simulink model "Cabinet_D"  (Simulink 7.6)
settings: Solver=ode45  StartTime=0.0  StopTime=1000  RelTol=1e-3
values from neighbouring files (symbols this model uses):
  R = 25    [ParametersCabinet_D.m]
  sb = 5.67*(10^-8)    (= 5.67e-08)    [ParametersCabinet_D.m]
  T_amb = 296    [ParametersCabinet_D.m]
undefined symbols (not defined in the file or in its folder): CNC, Job, magnitude
libraries: simulink x1
settings Model: Creator=conid  LastModifiedBy=conid

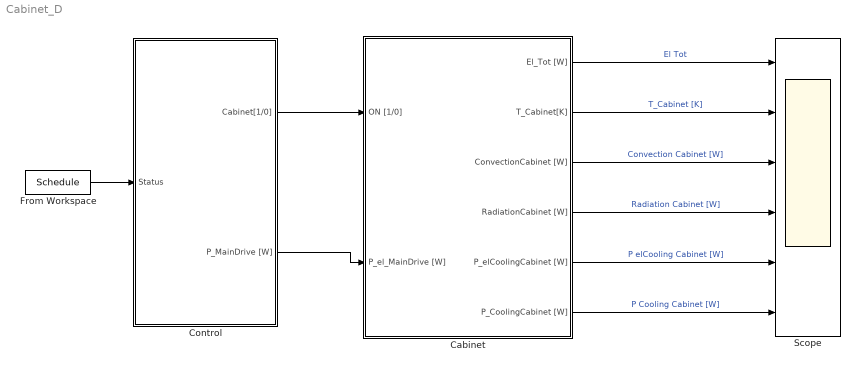
== system Cabinet_D ==
  Cabinet : Subsystem  TreatAsAtomicUnit=on
  Control : Subsystem  TreatAsAtomicUnit=on  mask{Cabinet=[0 1 1 1 1], Job=Job}
      mask prompts: Job "Job Struct"
      mask help:
      | Controls the components of the machine:
      |
      | Status:
      |     0. Off
      |     1. Standby
      |     2. Warmup
      |     3. Setting
      |     4. Machining
      |
      | If the status is machining, the job defined as
      |     - Job.time
      |     - Job.omega_dem
      |     - Job.M_dem
      | will be runned, and repeated.
      mask TabNameString: Status,Job
  From Workspace : FromWorkspace  VariableName=Schedule  SampleTime=0  Interpolate=off  OutputAfterFinalValue=Holding final value
  Scope : Scope  NumInputPorts=6
      settings: YMin=-5~-5~-5~-5~-5~-5  YMax=5~5~5~5~5~5  SaveName=Scp_Cabinet
  wires:
  Cabinet/1(El_Tot [W]) -> Scope/1  "El Tot"
  Cabinet/2(T_Cabinet[K]) -> Scope/2  "T_Cabinet [K]"
  Cabinet/3(ConvectionCabinet [W]) -> Scope/3  "Convection Cabinet [W]"
  Cabinet/4(RadiationCabinet [W]) -> Scope/4  "Radiation Cabinet [W]"
  Cabinet/5(P_elCoolingCabinet [W]) -> Scope/5  "P elCooling Cabinet [W]"
  Cabinet/6(P_CoolingCabinet [W]) -> Scope/6  "P Cooling Cabinet [W]"
  From Workspace/1 -> Control/1(Status)
  Control/1(Cabinet[1/0]) -> Cabinet/1(ON [1/0])
  Control/2(P_MainDrive [W]) -> Cabinet/2(P_el_MainDrive [W])

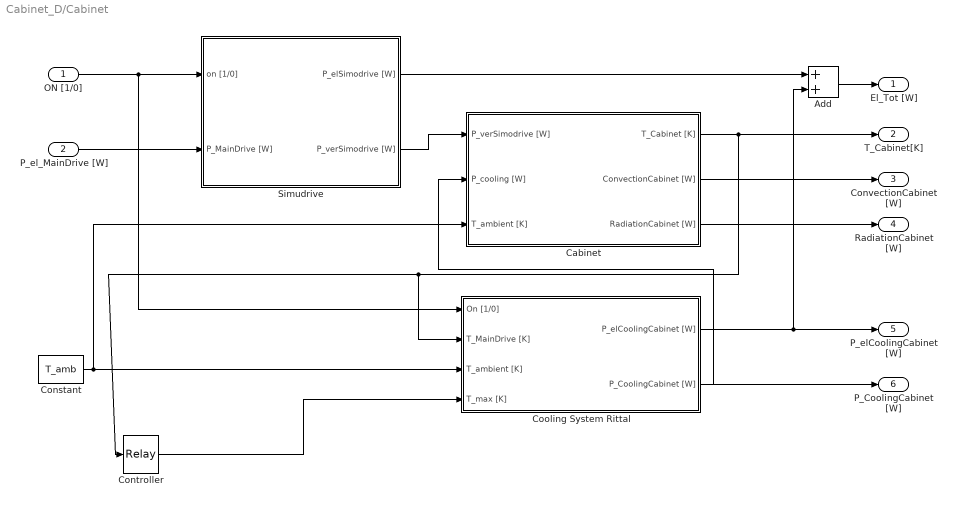
== system Cabinet_D/Cabinet ==
  ON [1/0] : Inport
  P_el_MainDrive [W] : Inport  Port=2
  Add : Sum
  Cabinet : Subsystem
  Constant : Constant  Value=T_amb
  Controller : Relay  OnSwitchValue=CNC.Cooling.Tmax  OffSwitchValue=CNC.Cooling.Tmin
  Cooling System Rittal : Subsystem
  Simudrive : Subsystem
  El_Tot [W] : Outport
  T_Cabinet[K] : Outport  Port=2
  ConvectionCabinet [W] : Outport  Port=3
  RadiationCabinet [W] : Outport  Port=4
  P_elCoolingCabinet [W] : Outport  Port=5
  P_CoolingCabinet [W] : Outport  Port=6
  wires:
  Cabinet/1(T_Cabinet [K]) -> Controller/1, Cooling System Rittal/2(T_MainDrive [K]), T_Cabinet[K]/1
  Constant/1 -> Cooling System Rittal/3(T_ambient [K]), Cabinet/3(T_ambient [K])
  Cooling System Rittal/2(P_CoolingCabinet [W]) -> Cabinet/2(P_cooling [W]), P_CoolingCabinet [W]/1
  Cabinet/2(ConvectionCabinet [W]) -> ConvectionCabinet [W]/1
  Cabinet/3(RadiationCabinet [W]) -> RadiationCabinet [W]/1
  Cooling System Rittal/1(P_elCoolingCabinet [W]) -> P_elCoolingCabinet [W]/1, Add/2
  P_el_MainDrive [W]/1 -> Simudrive/2(P_MainDrive [W])
  ON [1/0]/1 -> Simudrive/1(on [1/0]), Cooling System Rittal/1(On [1/0])
  Simudrive/2(P_verSimodrive [W]) -> Cabinet/1(P_verSimodrive [W])
  Simudrive/1(P_elSimodrive [W]) -> Add/1
  Controller/1 -> Cooling System Rittal/4(T_max [K])
  Add/1 -> El_Tot [W]/1

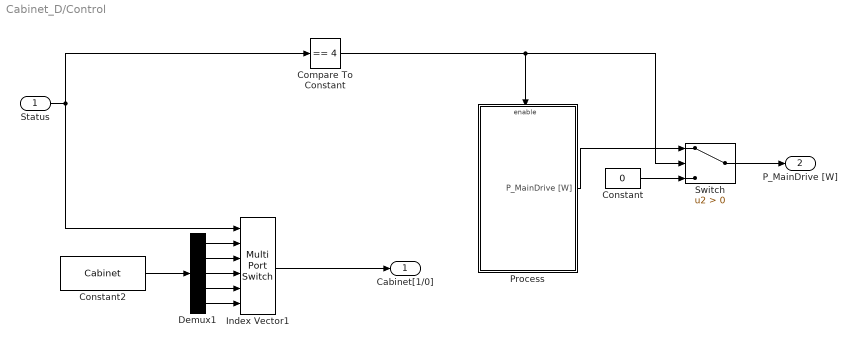
== system Cabinet_D/Control ==
  Status : Inport
  Compare To Constant : simulink/Logic and Bit Operations/Compare To Constant  SystemSampleTime=-1  relop===  const=4  LogicOutDataTypeMode=uint8
  Constant : Constant  Value=0
  Constant2 : Constant  Value=Cabinet
  Demux1 : Demux  Outputs=5
  Index Vector1 : MultiPortSwitch  DataPortOrder=Zero-based contiguous  Inputs=5  zeroidx=on
  Process : Subsystem  TreatAsAtomicUnit=on
  Switch : Switch  Criteria=u2 > Threshold
  Cabinet[1/0] : Outport
  P_MainDrive [W] : Outport  Port=2
  wires:
  Status/1 -> Compare To Constant/1, Index Vector1/1
  Demux1/1 -> Index Vector1/2
  Demux1/2 -> Index Vector1/3
  Demux1/3 -> Index Vector1/4
  Demux1/4 -> Index Vector1/5
  Demux1/5 -> Index Vector1/6
  Index Vector1/1 -> Cabinet[1/0]/1
  Compare To Constant/1 -> Process/Enable, Switch/2
  Process/1(P_MainDrive [W]) -> Switch/1
  Constant/1 -> Switch/3
  Switch/1 -> P_MainDrive [W]/1
  Constant2/1 -> Demux1/1

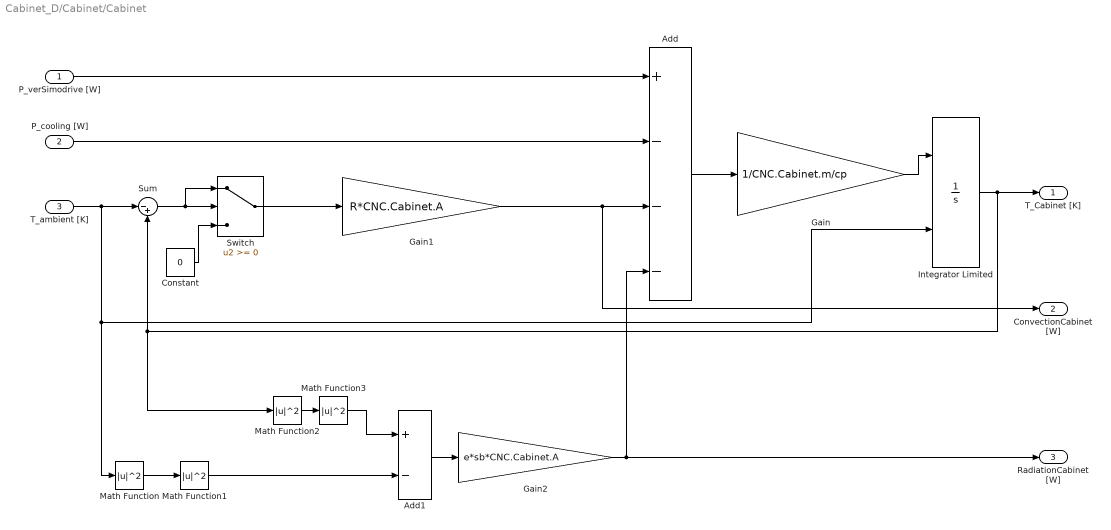
== system Cabinet_D/Cabinet/Cabinet ==
  P_verSimodrive [W] : Inport
  P_cooling [W] : Inport  Port=2
  T_ambient [K] : Inport  Port=3
  Add : Sum  Inputs=+---
  Add1 : Sum  Inputs=+-
  Constant : Constant  Value=0
  Gain : Gain  Gain=1/CNC.Cabinet.m/cp
  Gain1 : Gain  Gain=R*CNC.Cabinet.A
  Gain2 : Gain  Gain=e*sb*CNC.Cabinet.A
  Integrator Limited : Integrator  InitialConditionSource=external  LimitOutput=on
  Math Function{,1..3} (4 alike) : Math  Operator=magnitude^2  SaturateOnIntegerOverflow=on
  Sum : Sum  Inputs=|-+
  Switch : Switch
  T_Cabinet [K] : Outport
  ConvectionCabinet [W] : Outport  Port=2
  RadiationCabinet [W] : Outport  Port=3
  wires:
  P_verSimodrive [W]/1 -> Add/1
  Gain/1 -> Integrator Limited/1
  Gain1/1 -> ConvectionCabinet [W]/1, Add/3
  Integrator Limited/1 -> T_Cabinet [K]/1, Sum/2, Math Function2/1
  Add/1 -> Gain/1
  Math Function/1 -> Math Function1/1
  Gain2/1 -> RadiationCabinet [W]/1, Add/4
  P_cooling [W]/1 -> Add/2
  T_ambient [K]/1 -> Sum/1, Integrator Limited/2, Math Function/1
  Sum/1 -> Switch/2, Switch/1
  Constant/1 -> Switch/3
  Math Function2/1 -> Math Function3/1
  Add1/1 -> Gain2/1
  Math Function3/1 -> Add1/1
  Math Function1/1 -> Add1/2
  Switch/1 -> Gain1/1

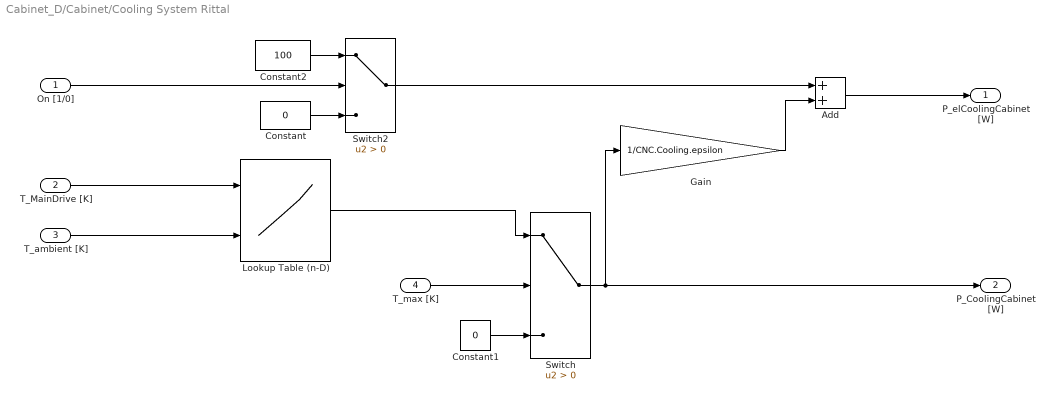
== system Cabinet_D/Cabinet/Cooling System Rittal ==
  On [1/0] : Inport
  T_MainDrive [K] : Inport  Port=2
  T_ambient [K] : Inport  Port=3
  T_max [K] : Inport  Port=4
  Add : Sum
  Constant : Constant  Value=0
  Constant1 : Constant  Value=0
  Constant2 : Constant  Value=100
  Gain : Gain  Gain=1/CNC.Cooling.epsilon
  Lookup Table (n-D) : Lookup_n-D  BreakpointsForDimension1=CNC.Cooling.T_int  BreakpointsForDimension2=CNC.Cooling.T_ext  Table=CNC.Cooling.Qdot  InterpMethod=Cubic spline  InputSameDT=on
  Switch : Switch  Criteria=u2 > Threshold
  Switch2 : Switch  Criteria=u2 > Threshold
  P_elCoolingCabinet [W] : Outport
  P_CoolingCabinet [W] : Outport  Port=2
  wires:
  Lookup Table (n-D)/1 -> Switch/1
  Switch/1 -> P_CoolingCabinet [W]/1, Gain/1
  On [1/0]/1 -> Switch2/2
  Constant/1 -> Switch2/3
  Constant2/1 -> Switch2/1
  Switch2/1 -> Add/1
  Add/1 -> P_elCoolingCabinet [W]/1
  Constant1/1 -> Switch/3
  T_ambient [K]/1 -> Lookup Table (n-D)/2
  T_MainDrive [K]/1 -> Lookup Table (n-D)/1
  Gain/1 -> Add/2
  T_max [K]/1 -> Switch/2

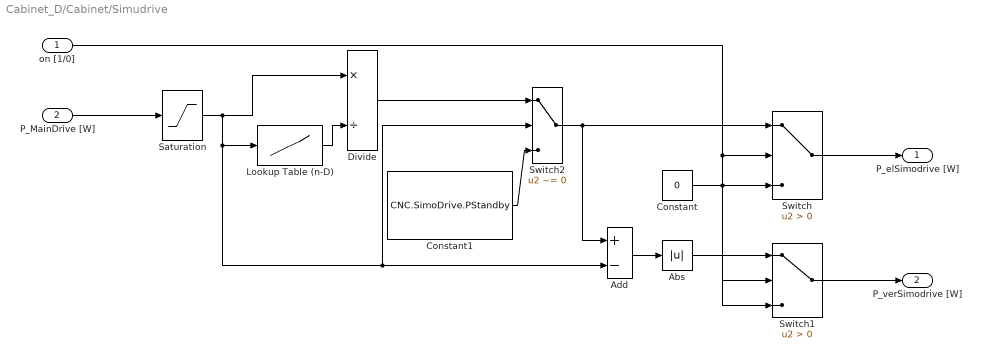
== system Cabinet_D/Cabinet/Simudrive ==
  on [1/0] : Inport
  P_MainDrive [W] : Inport  Port=2
  Abs : Abs
  Add : Sum  Inputs=+-
  Constant : Constant  Value=0
  Constant1 : Constant  Value=CNC.SimoDrive.PStandby
  Divide : Product  Inputs=*/
  Lookup Table (n-D) : Lookup_n-D  NumberOfTableDimensions=1  BreakpointsForDimension1=CNC.SimoDrive.OpPointsP  Table=CNC.SimoDrive.OpPointsEta  InputSameDT=on
  Saturation : Saturate  UpperLimit=Inf  LowerLimit=-Inf
  Switch : Switch  Criteria=u2 > Threshold
  Switch1 : Switch  Criteria=u2 > Threshold
  Switch2 : Switch  Criteria=u2 ~= 0
  P_elSimodrive [W] : Outport
  P_verSimodrive [W] : Outport  Port=2
  wires:
  Switch1/1 -> P_verSimodrive [W]/1
  Switch/1 -> P_elSimodrive [W]/1
  Abs/1 -> Switch1/1
  Constant/1 -> Switch/3, Switch1/3
  Add/1 -> Abs/1
  Switch2/1 -> Switch/1, Add/1
  P_MainDrive [W]/1 -> Saturation/1
  Lookup Table (n-D)/1 -> Divide/2
  Divide/1 -> Switch2/1
  Constant1/1 -> Switch2/3
  Saturation/1 -> Divide/1, Add/2, Switch2/2, Lookup Table (n-D)/1
  on [1/0]/1 -> Switch/2, Switch1/2

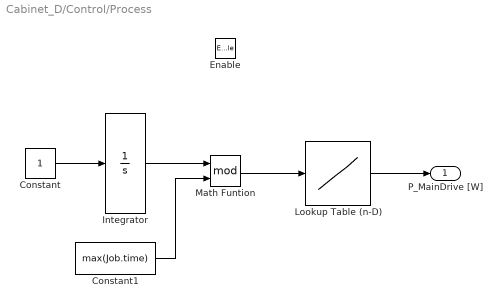
== system Cabinet_D/Control/Process ==
  Enable : EnablePort
  Constant : Constant
  Constant1 : Constant  Value=max(Job.time)
  Integrator : Integrator
  Lookup Table (n-D) : Lookup_n-D  NumberOfTableDimensions=1  BreakpointsForDimension1=Job.time  Table=Job.P_MainDrive  InterpMethod=None - Flat  ExtrapMethod=None - Clip  InputSameDT=on
  Math Funtion : Math  Operator=mod  SaturateOnIntegerOverflow=on
  P_MainDrive [W] : Outport
  wires:
  Constant/1 -> Integrator/1
  Integrator/1 -> Math Funtion/1
  Math Funtion/1 -> Lookup Table (n-D)/1
  Lookup Table (n-D)/1 -> P_MainDrive [W]/1
  Constant1/1 -> Math Funtion/2
